simulink model "Punto5"  (R2024b)
settings: Solver=VariableStepAuto  StartTime=0.0  StopTime=10  RelTol=1e-3
settings Model: Creator=Andres Felipe  LastModifiedBy=Andres Felipe

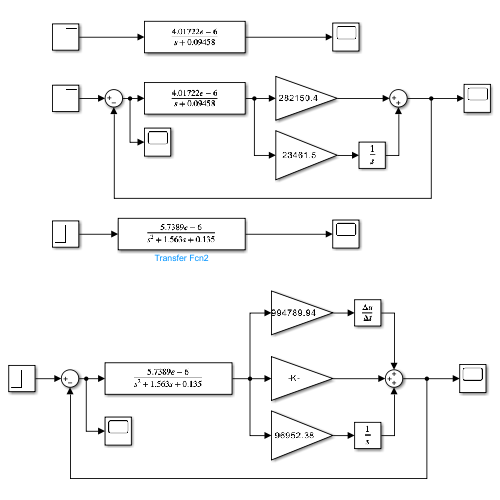
[thumbnail: Simulink's stored preview of the top-level diagram]
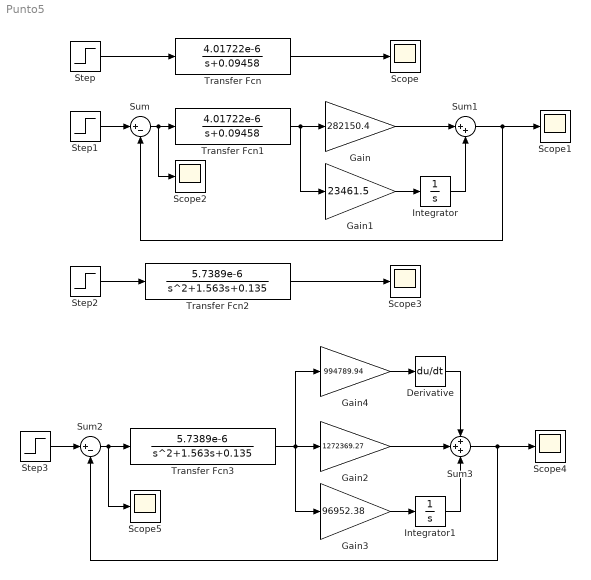
== system Punto5 ==
  Derivative : Derivative
  Gain : Gain  Gain=282150.4
  Gain1 : Gain  Gain=23461.5
  Gain2 : Gain  Gain=1272369.27
  Gain3 : Gain  Gain=96952.38
  Gain4 : Gain  Gain=994789.94
  Integrator : Integrator
  Integrator1 : Integrator
  Scope{,1..5} (6 alike) : Scope
  Step{,1..3} (4 alike) : Step  Time=0  SampleTime=0
  Sum : Sum  Inputs=|+-
  Sum1 : Sum  Inputs=|++
  Sum2 : Sum  Inputs=|+-
  Sum3 : Sum  Inputs=+++
  Transfer Fcn : TransferFcn  Numerator=[4.01722e-6]  Denominator=[1 0.09458]
  Transfer Fcn1 : TransferFcn  Numerator=[4.01722e-6]  Denominator=[1 0.09458]
  Transfer Fcn2 : TransferFcn  Numerator=[5.7389e-6]  Denominator=[1 1.563 0.135]
  Transfer Fcn3 : TransferFcn  Numerator=[5.7389e-6]  Denominator=[1 1.563 0.135]
  wires:
  Transfer Fcn/1 -> Scope/1
  Step/1 -> Transfer Fcn/1
  Sum/1 -> Scope2/1, Transfer Fcn1/1
  Step1/1 -> Sum/1
  Sum1/1 -> Sum/2, Scope1/1
  Transfer Fcn1/1 -> Gain1/1, Gain/1
  Gain1/1 -> Integrator/1
  Gain/1 -> Sum1/1
  Integrator/1 -> Sum1/2
  Transfer Fcn2/1 -> Scope3/1
  Step2/1 -> Transfer Fcn2/1
  Gain3/1 -> Integrator1/1
  Sum3/1 -> Sum2/2, Scope4/1
  Step3/1 -> Sum2/1
  Sum2/1 -> Transfer Fcn3/1, Scope5/1
  Transfer Fcn3/1 -> Gain3/1, Gain2/1, Gain4/1
  Gain4/1 -> Derivative/1
  Integrator1/1 -> Sum3/3
  Gain2/1 -> Sum3/2
  Derivative/1 -> Sum3/1
